simulink model "aileron_input"  (R2017a)
settings: Solver=VariableStepAuto  StartTime=0.0  StopTime=20  RelTol=1e-3
settings Model: Creator=ohanes  LastModifiedBy=ohanes

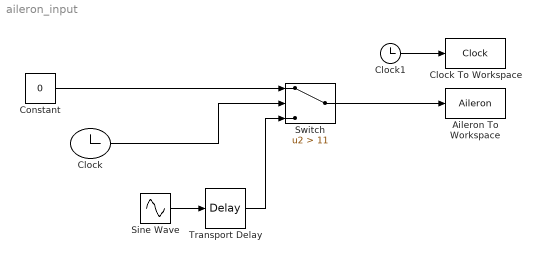
== system aileron_input ==
  Aileron To Workspace : ToWorkspace  VariableName=Aileron  SampleTime=-1
  Clock : Clock
  "Clock To Workspace " : ToWorkspace  VariableName=Clock  SampleTime=-1
  Clock1 : Clock
  Constant : Constant  Value=0
  Sine Wave : Sin  Amplitude=30  SampleTime=0
      settings: AttributesFormatString=Aileron Input
  Switch : Switch  Criteria=u2 > Threshold  Threshold=11
  Transport Delay : TransportDelay  DelayTime=5
  wires:
  Sine Wave/1 -> Transport Delay/1
  Clock/1 -> Switch/2
  Transport Delay/1 -> Switch/3
  Constant/1 -> Switch/1
  Switch/1 -> Aileron To Workspace/1
  Clock1/1 -> "Clock To Workspace "/1
